simulink model "NegativeFeedbackLoop"  (R2021a)
settings: Solver=VariableStepAuto  StartTime=0.0  StopTime=10.0  RelTol=1e-3
values from neighbouring files (symbols this model uses):
  A = [0 1 0 ... (first row only)    [IWP_SS_482Project.m]
  B = [0 ... (first row only)    [IWP_SS_482Project.m]
  C = eye(size(A))    [IWP_SS_482Project.m]
  D = zeros(size(C,1),size(B,2))    [IWP_SS_482Project.m]
  K = place(A,B,V)    [IWP_SS_482Project.m]
settings Model: Creator=Austin Mahannah  LastModifiedBy=Austin Mahannah

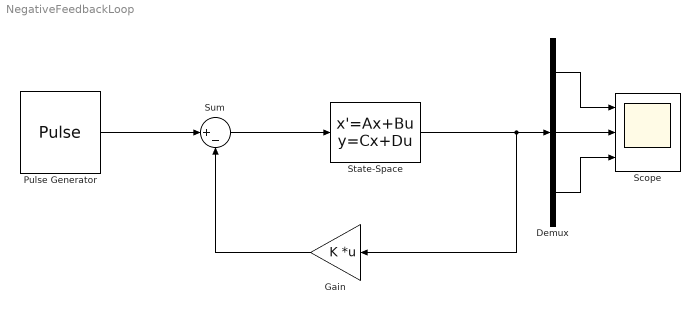
== system NegativeFeedbackLoop ==
  Demux : Demux  Outputs=3
  Gain : Gain  Gain=K  Multiplication=Matrix(K*u)
  Pulse Generator : DiscretePulseGenerator  PulseType=Time based  Period=1  PulseWidth=5
  Scope : Scope  NumInputPorts=3
  State-Space : StateSpace  A=A  B=B  C=C  D=D  InitialCondition=[-0.1 0 0]
  Sum : Sum  Inputs=|+-
  wires:
  Pulse Generator/1 -> Sum/1
  State-Space/1 -> Gain/1, Demux/1
  Demux/1 -> Scope/1
  Demux/2 -> Scope/2
  Demux/3 -> Scope/3
  Gain/1 -> Sum/2
  Sum/1 -> State-Space/1
